simulink model "AeroModel_Jaden"  (R2021a)
settings: Solver=ode4  StartTime=0.0  StopTime=10.0  FixedStep=0.0001  RelTol=1e-3
libraries: simulink_extras x4
settings Model: Creator=jadg1  LastModifiedBy=jadg1

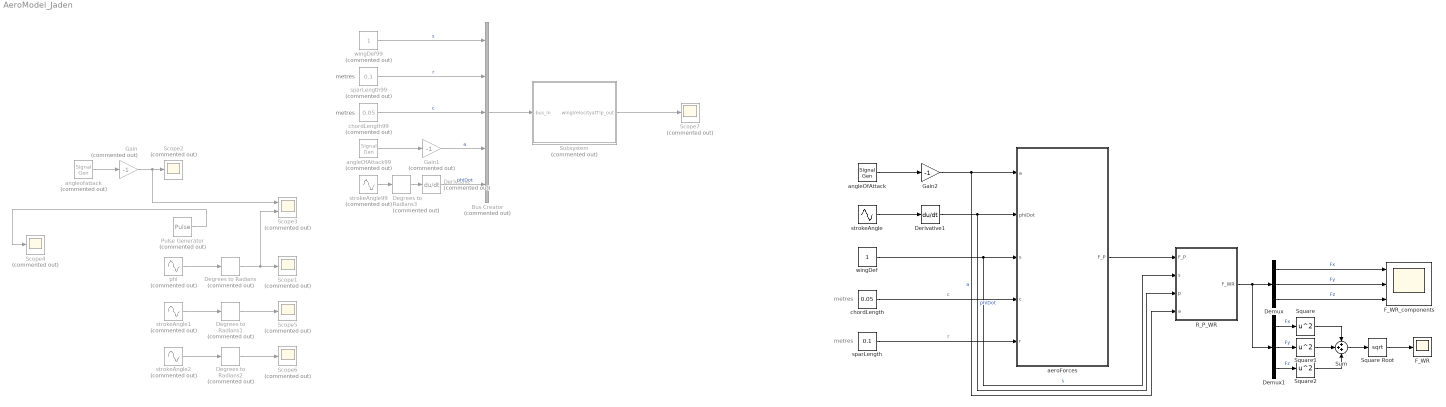
== system AeroModel_Jaden ==
  note: metres
  note: metres
  note: metres
  note: metres
  Bus Creator : BusCreator  Commented=on  Inputs=5
  Degrees to Radians{,1..3} (4 alike) : simulink_extras/Transformations/Degrees to Radians  Commented=on
  Demux : Demux  Outputs=3
  Demux1 : Demux  Outputs=3
  Derivative : Derivative  Commented=on
  Derivative1 : Derivative
  F_WR : Scope
  F_WR_components : Scope  NumInputPorts=3
  Gain : Gain  Commented=on  Gain=-1
  Gain1 : Gain  Commented=on  Gain=-1
  Gain2 : Gain  Gain=-1
  Pulse Generator : DiscretePulseGenerator  Commented=on  PulseType=Time based  Amplitude=pi()/4  Period=1/30  PulseWidth=50
  R_P_WR : MATLAB Function  TreatAsAtomicUnit=on
  Scope{1..2,4..7} (6 alike) : Scope  Commented=on
  Scope3 : Scope  Commented=on  NumInputPorts=2
  Square : Math  Operator=square  SaturateOnIntegerOverflow=on
  Square Root : Sqrt  SaturateOnIntegerOverflow=on
  Square1 : Math  Operator=square  SaturateOnIntegerOverflow=on
  Square2 : Math  Operator=square  SaturateOnIntegerOverflow=on
  Subsystem : Subsystem  Commented=on
  Sum : Sum  Inputs=+++
  aeroForces : MATLAB Function  TreatAsAtomicUnit=on
  angleOfAttack : SignalGenerator  WaveForm=square  Amplitude=pi()/4  Frequency=30
  angleOfAttack99 : SignalGenerator  Commented=on  WaveForm=square  Amplitude=pi()/4  Frequency=30
  angleofattack : SignalGenerator  Commented=on  WaveForm=square  Amplitude=pi()/4  Frequency=30
  chordLength : Constant  Value=0.05
  chordLength99 : Constant  Commented=on  Value=0.05
  phi : Sin  Commented=on  Amplitude=90  Frequency=188.5  Phase=pi()/2  SampleTime=0
  sparLength : Constant  Value=0.1
  sparLength99 : Constant  Commented=on  Value=0.1
  strokeAngle : Sin  Amplitude=pi()/2  Frequency=188.5  Phase=pi()/2  SampleTime=0
  strokeAngle1 : Sin  Commented=on  Amplitude=90  Frequency=188.5  SampleTime=0
  strokeAngle2 : Sin  Commented=on  Amplitude=90  Frequency=50  SampleTime=0
  strokeAngle99 : Sin  Commented=on  Amplitude=90  Frequency=188.5  Phase=pi()/2  SampleTime=0
  wingDef : Constant
  wingDef99 : Constant  Commented=on
  wires:
  aeroForces/1(F_P) -> R_P_WR/1(F_P)
  phi/1 -> Degrees to Radians/1
  Degrees to Radians/1 -> Scope3/2, Scope1/1
  angleofattack/1 -> Gain/1
  Pulse Generator/1 -> Scope4/1
  strokeAngle1/1 -> Degrees to Radians1/1
  Degrees to Radians1/1 -> Scope5/1
  strokeAngle2/1 -> Degrees to Radians2/1
  Degrees to Radians2/1 -> Scope6/1
  Gain/1 -> Scope3/1, Scope2/1
  Bus Creator/1 -> Subsystem/1(bus_in)
  wingDef99/1 -> Bus Creator/1  "s"
  sparLength99/1 -> Bus Creator/2  "r"
  chordLength99/1 -> Bus Creator/3  "c"
  angleOfAttack99/1 -> Gain1/1
  Gain1/1 -> Bus Creator/4  "a"
  strokeAngle99/1 -> Degrees to Radians3/1
  Degrees to Radians3/1 -> Derivative/1
  Derivative/1 -> Bus Creator/5  "phiDot"
  Subsystem/1(wingVelocityatTip_out) -> Scope7/1
  chordLength/1 -> aeroForces/4(c)  "c"
  strokeAngle/1 -> Derivative1/1
  Derivative1/1 -> aeroForces/2(phiDot), R_P_WR/3(p)  "phiDot"
  sparLength/1 -> aeroForces/5(r)  "r"
  wingDef/1 -> R_P_WR/2(s), aeroForces/3(s)  "s"
  angleOfAttack/1 -> Gain2/1
  Gain2/1 -> aeroForces/1(a), R_P_WR/4(a)  "a"
  R_P_WR/1(F_WR) -> Demux1/1, Demux/1
  Demux/1 -> F_WR_components/1  "Fx"
  Demux/2 -> F_WR_components/2  "Fy"
  Demux/3 -> F_WR_components/3  "Fz"
  Demux1/1 -> Square/1  "Fx"
  Demux1/2 -> Square1/1  "Fy"
  Demux1/3 -> Square2/1  "Fz"
  Square1/1 -> Sum/2
  Square/1 -> Sum/1
  Square2/1 -> Sum/3
  Sum/1 -> Square Root/1
  Square Root/1 -> F_WR/1

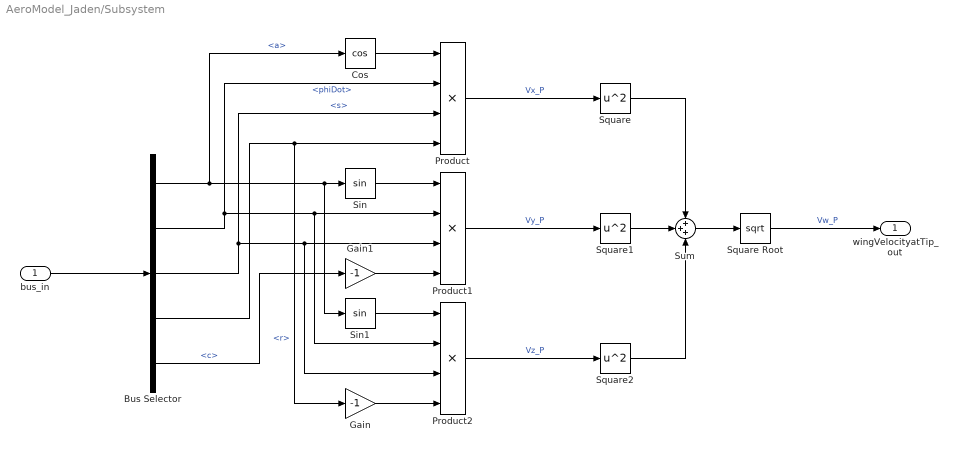
== system AeroModel_Jaden/Subsystem ==
  bus_in : Inport
  Bus Selector : BusSelector  OutputSignals=a,phiDot,s,r,c
  Cos : Trigonometry  Operator=cos
  Gain : Gain  Gain=-1
  Gain1 : Gain  Gain=-1
  Product : Product  Inputs=4
  Product1 : Product  Inputs=4
  Product2 : Product  Inputs=4
  Sin : Trigonometry
  Sin1 : Trigonometry
  Square : Math  Operator=square  SaturateOnIntegerOverflow=on
  Square Root : Sqrt  SaturateOnIntegerOverflow=on
  Square1 : Math  Operator=square  SaturateOnIntegerOverflow=on
  Square2 : Math  Operator=square  SaturateOnIntegerOverflow=on
  Sum : Sum  Inputs=+++
  wingVelocityatTip_out : Outport
  wires:
  Square Root/1 -> wingVelocityatTip_out/1  "Vw_P"
  bus_in/1 -> Bus Selector/1
  Bus Selector/1 -> Sin1/1, Sin/1, Cos/1  "<a>"
  Bus Selector/3 -> Product/3, Product2/3, Product1/3  "<s>"
  Bus Selector/4 -> Product/4, Gain/1  "<r>"
  Bus Selector/5 -> Gain1/1  "<c>"
  Cos/1 -> Product/1
  Bus Selector/2 -> Product2/2, Product1/2, Product/2  "<phiDot>"
  Sin/1 -> Product1/1
  Sin1/1 -> Product2/1
  Gain/1 -> Product2/4
  Gain1/1 -> Product1/4
  Product2/1 -> Square2/1  "Vz_P"
  Product1/1 -> Square1/1  "Vy_P"
  Product/1 -> Square/1  "Vx_P"
  Square1/1 -> Sum/2
  Square/1 -> Sum/1
  Square2/1 -> Sum/3
  Sum/1 -> Square Root/1

== matlab function AeroModel_Jaden/R_P_WR ==
  data: F_P input; F_WR output; s input; p input; a input
function F_WR = rotateForces(F_P,s,p,a)

F_WR = zeros(3,1);

R_P_WR = [  
            cos(s*p)*cos(a)      sin(s*p)        -cos(s*p)*sin(a)     ;
           -sin(s*p)*cos(a)      cos(s*p)         sin(s*p)*sin(a)     ;
                 sin(a)              0                  cos(a)        ;
         ];

F_WR = R_P_WR * F_P;     

end

== matlab function AeroModel_Jaden/aeroForces ==
  data: a input; F_P output; phiDot input; s input; c input; r input
function F_P = aeroForces(a,phiDot,s,c,r)

psi = 0;

% Declare sizes
F_P = zeros(3,1);

theta = -a;

p = 1.225; % density of air in kg/m^3

cL = 1.58*sin((2.13*a)-(7.2*(pi()/180))) + 0.225;

cD = 1.92 - 1.55*cos((2.04*a)-(9.82*(pi()/180)));

expr = (((cos(a)^2)*(c^3)*r)/3) - ((c^3)*r)/3 - ((r^3)*c)/3;

Fx_P = (-1/2)*cos(theta)*sign(a)*p*(phiDot^2)*(s^2)*cL*expr + (1/2)*sin(theta)*p*(phiDot^2)*(s^2)*cD*expr;

Fy_P = (-1/2)*cos(psi)*sin(theta)*sign(a)*p*(phiDot^2)*(s^2)*cL*expr - (1/2)*cos(psi)*cos(theta)*p*(phiDot^2)*(s^2)*cD*expr;

Fz_P = (1/2)*sin(psi)*sin(theta)*sign(a)*p*(phiDot^2)*(s^2)*cL*expr + (1/2)*sin(psi)*cos(theta)*p*(phiDot^2)*(s^2)*cD*expr;

F_P = [ Fx_P ;
        Fy_P ; 
        Fz_P ; ];

end
